simulink model "chap2_2sim"  (Simulink 6.3)
settings: Solver=ode45  StartTime=0.0  StopTime=2000  RelTol=1e-3
settings Model: Creator=hp  LastModifiedBy=Administrator
settings DataIOCC: SignalLoggingName=sigsOut
settings OptimizationCC: InlineInvariantSignals=on
settings DebuggingCC: SolverPrmCheckMsg=none
settings HardwareCC: TargetUnknown=on

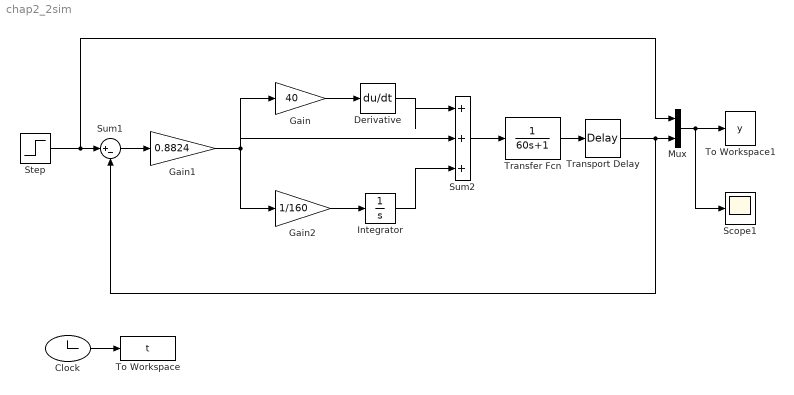
== system chap2_2sim ==
  Clock : Clock
  Derivative : Derivative
  Gain : Gain  Gain=40  SaturateOnIntegerOverflow=on
  Gain1 : Gain  Gain=0.8824  SaturateOnIntegerOverflow=on
  Gain2 : Gain  Gain=1/160  SaturateOnIntegerOverflow=on
  Integrator : Integrator
  Mux : Mux  Inputs=2
  Scope1 : Scope
  Step : Step  Time=0  SampleTime=0
  Sum1 : Sum  Inputs=|+-  SaturateOnIntegerOverflow=on
  Sum2 : Sum  Inputs=|+++  SaturateOnIntegerOverflow=on
  To Workspace : ToWorkspace  VariableName=t  SampleTime=-1  SaveFormat=Array
  To Workspace1 : ToWorkspace  VariableName=y  SampleTime=-1  SaveFormat=Array
  Transfer Fcn : TransferFcn  Denominator=[60 1]
  Transport Delay : TransportDelay  DelayTime=80
  wires:
  Step/1 -> Sum1/1, Mux/1
  Sum1/1 -> Gain1/1
  Sum2/1 -> Transfer Fcn/1
  Transfer Fcn/1 -> Transport Delay/1
  Transport Delay/1 -> Sum1/2, Mux/2
  Gain1/1 -> Gain/1, Sum2/2, Gain2/1
  Gain/1 -> Derivative/1
  Gain2/1 -> Integrator/1
  Integrator/1 -> Sum2/3
  Clock/1 -> To Workspace/1
  Mux/1 -> To Workspace1/1, Scope1/1
  Derivative/1 -> Sum2/1
